simulink model "Controlled_DoubleTank_Socket"  (R2021b)
settings: Solver=VariableStepAuto  StartTime=0.0  StopTime=200  RelTol=1e-3
values from neighbouring files (symbols this model uses):
  A = [0.967743748526  0; 0.031730333008  0.967743748526]    [Dados_Tanques.mat]    (also in double_tank_simu.m = sysd.A; nma_simplex.m = tab(1:nRow-1,1:nCol-1); nma_simplex_2.m = tab(1:nRow-1,1:nCol-1))
  a1 = 0.17795237427    [Dados_Tanques.mat]    (also in double_tank_simu.m)
  A1 = 15.5179165474    [Dados_Tanques.mat]    (also in double_tank_simu.m)
  A2 = 15.5179165474    [Dados_Tanques.mat]    (also in double_tank_simu.m)
  a2 = 0.17795237427    [Dados_Tanques.mat]    (also in double_tank_simu.m)
  B = [0.104604453049 0.0017055116738]    [Dados_Tanques.mat]    (also in double_tank_simu.m = sysd.B)
  g = 981    [Dados_Tanques.mat]    (also in double_tank_simu.m)
  Gv = [1 -1 0 0 0.0316763086938 -0.0316763086938 0.0610064360648 -0.0610064360648 0.0878578258116 -0.0878578258116 0.112163466595 -0.112163466595 ... (32 elements, 16x2)]    [Dados_Tanques.mat]
  km = 3.3    [Dados_Tanques.mat]    (also in double_tank_simu.m = 4.1)
  phi = [2.74907887757 9.25092112243]    [Dados_Tanques.mat]    (also in double_tank_simu.m = [(12-ueq) ueq]')
  rhov = [15 15 15 15 14.8404669643 14.8293968766 14.6652011254 14.6221983313 14.4769073428 14.3832726141 14.2782768412 14.1176408708 ... (16 elements, 16x1)]    [Dados_Tanques.mat]
  U = [1 -1]    [Dados_Tanques.mat]    (also in double_tank_simu.m = [1 -1]')
  ueq = 9.25092112243    [Dados_Tanques.mat]    (also in double_tank_simu.m = (a1/km)*sqrt(2*g*x1eq))
  x1eq = 15    [Dados_Tanques.mat]    (also in double_tank_simu.m = (1/(2*g))*((km*ueq)/a1)^2)
  x2eq = 15    [Dados_Tanques.mat]    (also in double_tank_simu.m)
undefined symbols (not defined in the file or in its folder): control
libraries: instrumentlib x2
settings Model: Creator=mathe  LastModifiedBy=mathe

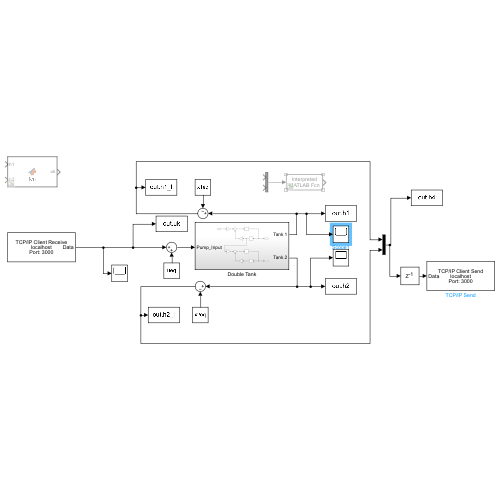
[thumbnail: Simulink's stored preview of the top-level diagram]
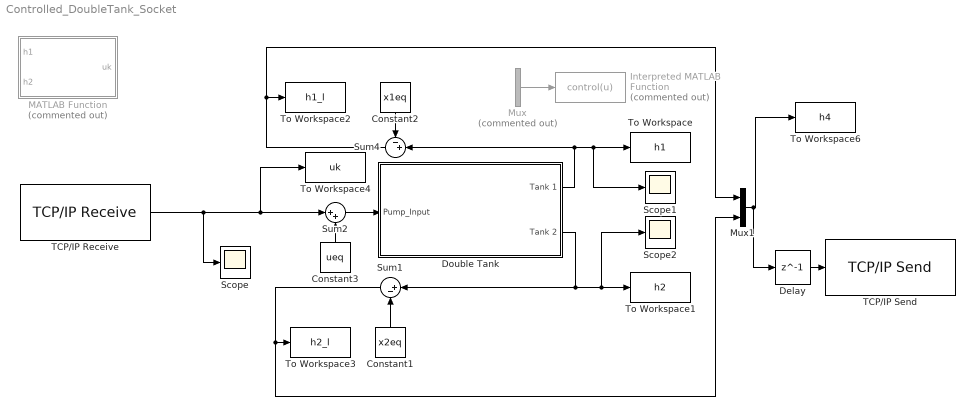
== system Controlled_DoubleTank_Socket ==
  Constant1 : Constant  Value=x2eq
  Constant2 : Constant  Value=x1eq
  Constant3 : Constant  Value=ueq
  Delay : Delay  DelayLength=1  InitialCondition=0
  Double Tank : Subsystem
  Interpreted MATLAB Function : MATLABFcn  Commented=on  MATLABFcn=control(u)
  MATLAB Function : MATLAB Function  Commented=on  TreatAsAtomicUnit=on
  Mux : Mux  Commented=on  Inputs=2
  Mux1 : Mux  Inputs=2
  Scope : Scope
  Scope1 : Scope
  Scope2 : Scope
  Sum1 : Sum  Inputs=|+-
  Sum2 : Sum  Inputs=|++
  Sum4 : Sum  Inputs=-+|
  TCP/IP Receive : instrumentlib/TCP//IP Receive  Priority=2  Host=localhost  Port=3000  DataSize=[ 1, 1 ]  DataType=double  ASCIIFormatting=%f  Terminator=LF  CustomTerminator=10  ByteOrder=big-endian  EnableBlockingMode=on  Timeout=200  SampleTime=0.1  SimulateUsing=Interpreted execution
  TCP/IP Send : instrumentlib/TCP//IP Send  Priority=1  Host=localhost  Port=3000  ByteOrder=big-endian  EnableBlockingMode=on  Timeout=500  TransferDelay=off  SimulateUsing=Interpreted execution
  To Workspace : ToWorkspace  VariableName=h1  SaveFormat=Timeseries  SampleTime=-1
  To Workspace1 : ToWorkspace  VariableName=h2  SaveFormat=Timeseries  SampleTime=-1
  To Workspace2 : ToWorkspace  VariableName=h1_l  SaveFormat=Timeseries  SampleTime=-1
  To Workspace3 : ToWorkspace  VariableName=h2_l  SaveFormat=Timeseries  SampleTime=-1
  To Workspace4 : ToWorkspace  VariableName=uk  SaveFormat=Timeseries  SampleTime=-1
  To Workspace6 : ToWorkspace  VariableName=h4  SaveFormat=Timeseries  SampleTime=-1
  wires:
  Sum1/1 -> To Workspace3/1, Mux1/2
  Double Tank/2(Tank 2) -> Scope2/1, To Workspace1/1, Sum1/1
  Constant1/1 -> Sum1/2
  Constant2/1 -> Sum4/1
  Sum2/1 -> Double Tank/1(Pump_Input)
  Constant3/1 -> Sum2/2
  Double Tank/1(Tank 1) -> Sum4/2, Scope1/1, To Workspace/1
  Mux/1 -> Interpreted MATLAB Function/1
  Mux1/1 -> Delay/1, To Workspace6/1
  Sum4/1 -> Mux1/1, To Workspace2/1
  TCP/IP Receive/1 -> To Workspace4/1, Sum2/1, Scope/1
  Delay/1 -> TCP/IP Send/1

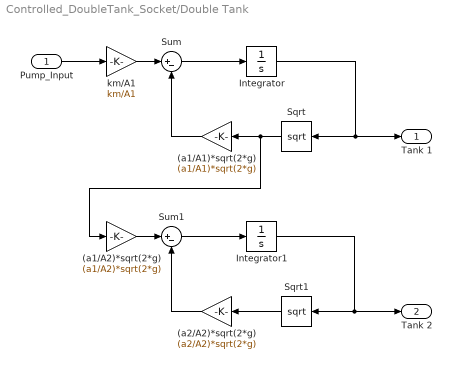
== system Controlled_DoubleTank_Socket/Double Tank ==
  Pump_Input : Inport
  (a1/A1)*sqrt(2*g) : Gain  Gain=(a1/A1)*sqrt(2*g)
  (a1/A2)*sqrt(2*g) : Gain  Gain=(a1/A2)*sqrt(2*g)
  (a2/A2)*sqrt(2*g) : Gain  Gain=(a2/A2)*sqrt(2*g)
  Integrator : Integrator  InitialCondition=15+1
  Integrator1 : Integrator  InitialCondition=15+1
  Sqrt : Sqrt  SaturateOnIntegerOverflow=on
  Sqrt1 : Sqrt  SaturateOnIntegerOverflow=on
  Sum : Sum  Inputs=|+-
  Sum1 : Sum  Inputs=|+-
  km/A1 : Gain  Gain=km/A1
  Tank 1 : Outport  VectorParamsAs1DForOutWhenUnconnected=off
  Tank 2 : Outport  Port=2  VectorParamsAs1DForOutWhenUnconnected=off
  wires:
  km/A1/1 -> Sum/1
  Integrator/1 -> Sqrt/1, Tank 1/1
  (a1/A2)*sqrt(2*g)/1 -> Sum1/1
  Sqrt/1 -> (a1/A2)*sqrt(2*g)/1, (a1/A1)*sqrt(2*g)/1
  Sum/1 -> Integrator/1
  (a2/A2)*sqrt(2*g)/1 -> Sum1/2
  Sum1/1 -> Integrator1/1
  (a1/A1)*sqrt(2*g)/1 -> Sum/2
  Sqrt1/1 -> (a2/A2)*sqrt(2*g)/1
  Pump_Input/1 -> km/A1/1
  Integrator1/1 -> Tank 2/1, Sqrt1/1

== matlab function Controlled_DoubleTank_Socket/MATLAB Function ==
  data: h1 input; uk output; h2 input; Gv parameter; B parameter; rhov parameter; U parameter; A parameter; phi parameter
%%%%%%%%%%%%%%%%%%%%%%%%%%%%%%%%%%%%
% STATIC STATE FEEDBACK CONTROLLER %
%%%%%%%%%%%%%%%%%%%%%%%%%%%%%%%%%%%%

function uk = fcn(h1, h2, Gv, B, rhov, U, A, phi)
    % hard-coded paramenters
    ncu = 1;
    nlu = 2;
    
    %coder.extrinsic('nma_simplex');
    xk = [h1 h2]';
    c = [zeros(ncu, 2) 1 -1  zeros(1,15)];
    Aa = [[Gv*B -Gv*B -rhov rhov; U -U zeros(nlu, 1) zeros(nlu, 1)] eye(15)];
    b = [-Gv*A*xk; phi];

    %====== NMA_SIMPLEX
    %===== validate_input(Aa,b,c);
    if ~ismatrix(Aa)
        error('A must be matrix');
    end
    
    if ~isvector(b)
        error('b must be vector');
    end
    if ~isvector(c)
        error('c must be vector');
    end
    
    [m,n]=size(Aa);
    if rank(Aa) <m
        error('Rank A must be equal to number of rows in A');
    end
    
    if length(b) ~= m
        error('b must have same size as number of rows of A');
    end
    if length(c) ~= n
        error('c must have same size as number of columns of A');
    end
    %===== end validate_input(Aa,b,c);

    %==== [Aa,b] = make_phase_one(Aa,b,debug);
    [m_aux,n_aux]              = size(Aa);
    tab                = zeros(m_aux+1,n_aux+m_aux+1);
    tab(1:m_aux,1:n_aux)       = Aa;
    tab(end,n_aux+1:end-1) = 1;
    tab(1:m_aux,end)       = b(:);
    tab(1:m_aux,n_aux+1:n_aux+m_aux)   = eye(m_aux);

    for i = 1:m_aux %now make all entries in bottom row zero
        tab(end,:) = tab(end,:)-tab(i,:);
    end

    %==== tab = simplex(tab(1:m,1:n+m),tab(1:m,end),tab(end,1:n+m),debug,'phase one');
    Aa_aux = tab(1:m,1:n+m);
    b_aux = tab(1:m,end);
    c_aux = tab(end,1:n+m);

    [m,n]        = size(Aa_aux);
    tab          = zeros(m+1,n+1);
    tab(1:m,1:n) = Aa_aux;
    tab(m+1,1:n) = c_aux(:);
    tab(1:m,end) = b_aux(:);

    keep_running = true;
    while keep_running
        
        if any(tab(end,1:n)<0)%check if there is negative cost coeff.
            [~,J] = min(tab(end,1:n)); %yes, find the most negative
            % now check if corresponding column is unbounded
            if all(tab(1:m,J)<=0) 
              error('problem unbounded. All entries <= 0 in column %d',J);
            %do row operations to make all entries in the column 0 
            %except pivot
            else 
                pivot_row = 0;
                min_found = inf;
                for i = 1:m
                    if tab(i,J)>0
                        tmp = tab(i,end)/tab(i,J);
                        if tmp < min_found
                            min_found = tmp;
                            pivot_row = i;
                        end
                    end
                end
                %normalize
                tab(pivot_row,:) = tab(pivot_row,:)/tab(pivot_row,J); 
                %now make all entries in J column zero.
                for i=1:m+1
                    if i ~= pivot_row
                        tab(i,:)=tab(i,:)-sign(tab(i,J))*...
                                    abs(tab(i,J))*tab(pivot_row,:);
                    end
                end
            end
        else
            keep_running=false;       
        end
    end
    %==== END tab = simplex(tab(1:m,1:n+m),tab(1:m,end),tab(end,1:n+m),debug,'phase one');

    Aa = tab(1:m_aux,1:n_aux);
    b = tab(1:m_aux,end);
    %==== end [Aa,b] = make_phase_one(Aa,b,debug);

    %==== tab = simplex(Aa,b,c,debug,'phase two')
    [m,n]        = size(Aa);
    tab          = zeros(m+1,n+1);
    tab(1:m,1:n) = Aa;
    tab(m+1,1:n) = c(:);
    tab(1:m,end) = b(:);

    keep_running = true;
    while keep_running
        
        if any(tab(end,1:n)<0)%check if there is negative cost coeff.
            [~,J] = min(tab(end,1:n)); %yes, find the most negative
            % now check if corresponding column is unbounded
            if all(tab(1:m,J)<=0) 
            error('problem unbounded. All entries <= 0 in column %d',J);
            %do row operations to make all entries in the column 0 
            %except pivot
            else 
                pivot_row = 0;
                min_found = inf;
                for i = 1:m
                    if tab(i,J)>0
                        tmp = tab(i,end)/tab(i,J);
                        if tmp < min_found
                            min_found = tmp;
                            pivot_row = i;
                        end
                    end
                end
                %normalize
                tab(pivot_row,:) = tab(pivot_row,:)/tab(pivot_row,J); 
                %now make all entries in J column zero.
                for i=1:m+1
                    if i ~= pivot_row
                        tab(i,:)=tab(i,:)-sign(tab(i,J))*...
                                    abs(tab(i,J))*tab(pivot_row,:);
                    end
                end
            end
        else
            keep_running=false;       
        end
    end
    %==== END tab = simplex(Aa,b,c,debug,'phase two')
    
    %==== sol = print_solution_vector(tab);
    [nRow,nCol] = size(tab);

    A = tab(1:nRow-1,1:nCol-1);
    b = tab(1:nRow-1,nCol);

    q = A ~= 0;
    q = find(sum(q,1)==1); %find all columns with one non-zero entry;

    sol = zeros(nCol-1,1); 

    for n=1:length(q)
        j = find(A(1:nRow-1,q(n))==1);
        if isempty(j)
         sol(q(n)) = 0;
        else
         sol(q(n)) = b(j); 
        end
    end
    %==== END sol = print_solution_vector(tab);
    %====== END NMA_SIMPLEX
    
    uk = sol(1) - sol(2);
end
